simulink model "inverted_pendulum_simulink_model"  (R2023b)
settings: Solver=VariableStepAuto  StartTime=0.0  StopTime=10.0  RelTol=1e-3
values from neighbouring files (symbols this model uses):
  K = place(A,B,Poles)    [Lqr_mass_spring_damper.m]    (also in N20_motor_closed_loop.m)
settings Model: Creator=sarth  LastModifiedBy=sarth

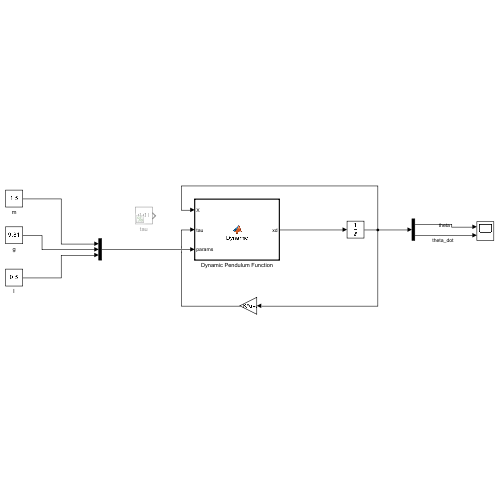
[thumbnail: Simulink's stored preview of the top-level diagram]
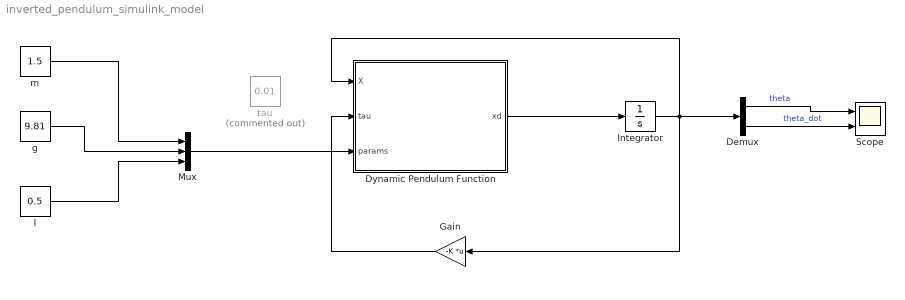
== system inverted_pendulum_simulink_model ==
  Demux : Demux  Outputs=2
  Dynamic Pendulum Function : MATLAB Function  TreatAsAtomicUnit=on
  Gain : Gain  Gain=-K  Multiplication=Matrix(K*u) (u vector)
  Integrator : Integrator  InitialCondition=[1;0]
  Mux : Mux  Inputs=3
  Scope : Scope  NumInputPorts=2
  g : Constant  Value=9.81
  l : Constant  Value=0.5
  m : Constant  Value=1.5
  tau : Constant  Commented=on  Value=0.01
  wires:
  Mux/1 -> Dynamic Pendulum Function/3(params)
  m/1 -> Mux/1
  g/1 -> Mux/2
  l/1 -> Mux/3
  Dynamic Pendulum Function/1(xd) -> Integrator/1
  Gain/1 -> Dynamic Pendulum Function/2(tau)
  Demux/1 -> Scope/1  "theta"
  Demux/2 -> Scope/2  "theta_dot"
  Integrator/1 -> Gain/1, Demux/1, Dynamic Pendulum Function/1(X)

== matlab function inverted_pendulum_simulink_model/Dynamic Pendulum Function ==
  data: X input; xd output; tau input; params input
function xd = Dynamic(X, tau, params)
m = params(1);
g = params(2);
l = params(3);

xd1 = X(2);
xd2 = ((1/m*l^2)*tau) - ((g/l)*sin(X(1)));

xd = [xd1; xd2];
